simulink model "testModel"  (R2016b)
settings: Solver=VariableStepAuto  StartTime=0.0  StopTime=10.0  RelTol=1e-3
undefined symbols (not defined in the file or in its folder): numGc
settings Model: Creator=Dai Luyao  LastModifiedBy=Dai Luyao

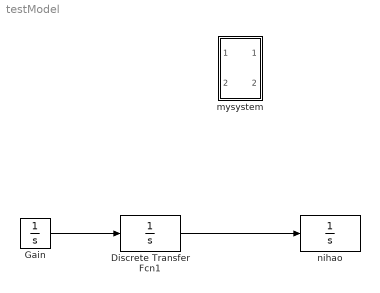
== system testModel ==
  Discrete Transfer Fcn1 : Integrator
  Gain : Integrator
  mysystem : Subsystem
  nihao : Integrator
  wires:
  Gain/1 -> Discrete Transfer Fcn1/1
  Discrete Transfer Fcn1/1 -> nihao/1

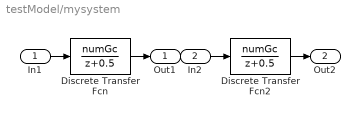
== system testModel/mysystem ==
  In1 : Inport
  In2 : Inport  Port=2
  Discrete Transfer Fcn : DiscreteTransferFcn  Numerator=numGc
  Discrete Transfer Fcn2 : DiscreteTransferFcn  Numerator=numGc
  Out1 : Outport
  Out2 : Outport  Port=2
  wires:
  In1/1 -> Discrete Transfer Fcn/1
  Discrete Transfer Fcn/1 -> Out1/1
  In2/1 -> Discrete Transfer Fcn2/1
  Discrete Transfer Fcn2/1 -> Out2/1
